simulink model "Control_APF7_nuevo_MicroLabBox"  (R2018b)
settings: Solver=FixedStepDiscrete  StartTime=0.0  StopTime=inf  FixedStep=Tm  RelTol=1e-3
PostLoadFcn:
  | , if any(exist('dsrtsu_mdlpostloadfcn', 'file') == [2, 3, 6]), try dsrtsu_mdlpostloadfcn('Execute', bdroot); catch fprintf('Error in PostLoadFcn (dsrtsu_mdlpostloadfcn) for model "%s":\n %s\n', bdroot, lasterr); end, end,
values from neighbouring files (symbols this model uses):
  e = den(1)    [parametrosAPF_nuevo.m]
  f = den(2)    [parametrosAPF_nuevo.m]
  g = den(3)    [parametrosAPF_nuevo.m]
  Ganancia_Ica = 2.6804*K    (= 26.804)    [parametrosAPF_nuevo.m]
  Ganancia_Icb = 2.7956*K    (= 27.956)    [parametrosAPF_nuevo.m]
  Ganancia_Icc = 2.7659*K    (= 27.659)    [parametrosAPF_nuevo.m]
  Ganancia_Ila = 2.7659*K    (= 27.659)    [parametrosAPF_nuevo.m]
  Ganancia_Ilb = 2.7659*K    (= 27.659)    [parametrosAPF_nuevo.m]
  Ganancia_Ilc = 2.7083*K    (= 27.083)    [parametrosAPF_nuevo.m]
  Ganancia_Vsa = 250.0    (= 250)    [parametrosAPF_nuevo.m]
  Ganancia_Vsb = 250.0    (= 250)    [parametrosAPF_nuevo.m]
  Ganancia_Vsc = 250.0    (= 250)    [parametrosAPF_nuevo.m]
  Ica_offset = 0.0    (= 0)    [parametrosAPF_nuevo.m]
  Icb_offset = 0.0    (= 0)    [parametrosAPF_nuevo.m]
  Icc_offset = 0.0    (= 0)    [parametrosAPF_nuevo.m]
  Ila_offset = 0.0    (= 0)    [parametrosAPF_nuevo.m]
  Ilb_offset = 0.0    (= 0)    [parametrosAPF_nuevo.m]
  Ilc_offset = 0.0    (= 0)    [parametrosAPF_nuevo.m]
  ki = 0.006    [parametrosAPF_nuevo.m]
  kp = 0.007    [parametrosAPF_nuevo.m]
  lamda = 0.02    [parametrosAPF_nuevo.m]
  Lc = 10e-3    (= 0.01)    [parametrosAPF_nuevo.m]
  Rc = 0.35    [parametrosAPF_nuevo.m]
  sat = 0    [parametrosAPF_nuevo.m]
  Ts = 1/10000    (= 0.0001)    [parametros.m]    (also in parametrosAPF_nuevo.m = 5.55555555556e-05)
  Vdc = 63.0    (= 63)    [parametrosAPF_nuevo.m]
  Vsa_offset = 1.507    [parametrosAPF_nuevo.m]
  Vsb_offset = 1.466    [parametrosAPF_nuevo.m]
  Vsc_offset = 1.495    [parametrosAPF_nuevo.m]
  x = num(1)    [parametrosAPF_nuevo.m]
  y = num(2)    [parametrosAPF_nuevo.m]
  z = num(3)    [parametrosAPF_nuevo.m]
libraries: rti1202lib_dio_class1 x20, rti1202lib_adc_class1 x12, RTITaskLibDemoLibInfo x2, simulink x1, rtitasklib x1
(part 1 of 4)
PreSaveFcn:
  | , if any(exist('dsmpb_private', 'file') == [2, 3, 6]), try, dsmpb_private('dsmpb_mdlclblib', 'PreSave', bdroot); catch, disp(lasterr); end, end,
CloseFcn:
  | , if any(exist('dsmpb_private', 'file') == [2, 3, 6]), try, dsmpb_private('dsmpb_mdlclblib', 'Close', bdroot); catch, disp(lasterr); end, end,
settings Model: DSRTSU_INTERNAL_RTI_VER=520  DSRTSU_INTERNAL_RTI_TYPE=rti1202  RTICANMMDATA=struct('GeneralSetupData',struct('modelroot',['C:\Users\DELL\Documents\Espinoza\APF 7Nuevo\Plantilla_Control_DMC_MicroLabBox'],'generalsettings',struct('filesettings',struct('destfolder',struct('Name','RTICANMM_FILES','Check',1),'buildfolder',struct('Name','.','Check',1),'AbsDestfolder',struct('Name',['C:\Users\DELL\Documents\Espinoza\APF 7Nuevo\Plantilla_Control_DMC_MicroLabBox\RTICANMM_FILES']),'AbsBuildfolder',struct('Name',['C:\Users\DELL\Documents\Espinoza\APF 7Nuevo\Plantilla_Control_DMC_MicroLabBox']))),'options',struct('addpaths',1,'rmpaths',1,'addtrcexclusion',logical(1),'cannavigator',struct('checkmonitoring',0),'show_usrtrc',0,'use_usrtrc',0),'advanced',struct('options',[1 1 1 1 1 1 1 1 1 1 1 1 1 1 1 1 1 1 1 1 1 1 1 1 1 1 1 1 1 1 1 1 1 1 1 1 1 1 1 1 1 1 1 1 1 1 1 1 1 1 1 1 1 1 1 1 1 1 1 1 1 1 1 1 1 1 1 1 1 1 1 1 1 1 1 1 1 1 1 1 1 1 1 1 1 1 1 1 1 1 1 1 1 1 1 1 1 1 1 1]),'MPSetup',{{}},'modelname','Control_APF7_nuevo_MicroLabBox','block','Control_APF7_nuevo_MicroLabBox'))  DSRTSU_INTERNAL_RTIFLEXRAYCONFIG=110  DSRTSU_INTERNAL_RTIFPGA=110  DSMPB_DATASERVER_ModelPortLibVersion1=8  DSMPB_DATASERVER_DataServerVersion1=6  DSMPB_DATASERVER_DataServerStreamVersion1=3  Creator=DELL  LastModifiedBy=DELL
settings OptimizationCC: BlockReduction=off  BufferReuse=off
settings HardwareCC: ProdBitPerPointer=32  ProdBitPerSizeT=32  ProdBitPerPtrDiffT=32  ProdLargestAtomicInteger=Integer  ProdEndianess=BigEndian  ProdWordSize=32  ProdHWDeviceType=Custom Processor->Custom  TargetIntDivRoundTo=Zero  TargetEndianess=BigEndian  TargetHWDeviceType=Custom Processor->Custom
settings SFSimCC: MATLABDynamicMemAlloc=off
settings RTWCC: SystemTargetFile=rti1202.tlc  MakeCommand=make_rti  TemplateMakefile=rti1202.tmf  Description=dSPACE DS1202 Hardware Platform
settings STFCustomTargetCC: ParMdlRefBuildCompliant=on  SystemTargetFile=rti1202.tlc
settings GRTTargetCC: TargetLangStandard=C89/C90 (ANSI)  CompOptLevelCompliant=off  ConcurrentExecutionCompliant=off  CombineOutputUpdateFcns=off  MatFileLogging=off  CPPClassGenCompliant=off  UseToolchainInfoCompliant=off  RTWCAPISignals=on

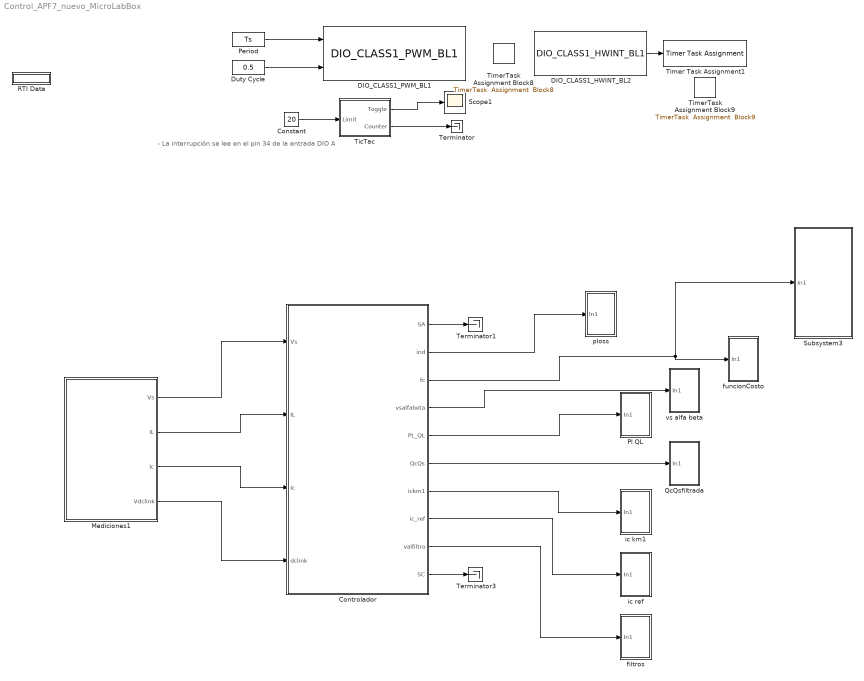
== system Control_APF7_nuevo_MicroLabBox ==
  note: - La interrupción se lee en el pin 34 de la entrada DIO A
  Constant : Constant  Value=20
  Controlador : Subsystem
  DIO_CLASS1_HWINT_BL2 : rti1202lib_dio_class1/DIO_CLASS1_HWINT_BL1  DSProperties=struct('RTI',struct('Version',uint32(2),'BlockType',struct('isSLSource',uint8(1),'isSLSink',uint8(0),'isHWSource',uint8(0),'isHWSink',uint8(0),'isSetup',uint8(0),'isInline',uint8(1),'isNonInline',uint8(0),'isInterrupt',uint8(1),'isChannelwise',uint8(0)),'IOBoardType',{{'DS120X','STD','DIOC1'}},'UnitType','DSTASKTOOL','Identifier','HWINT','DialogType','ML','BlockSet','NONE','SlaveProcessor','NONE'))  RTIBlockInterface=struct('OutputPortsActive',1,'OutputPortsWidth',int32(1),'OutputPortsName',{{'Interrupt'}},'FunctionCall',uint32(0),'DialogFcn','rti120xstddioc1hwintgui','InitLevel',3,'BlockDisplay',{{['DIO CL1 HWINT\nIdentifier: PWM\nPort: 3\nChannel: 1\nInterrupt: Falling edge'],'center'}},'IconTransparency','on','BlockName',struct('Token',{{'DIO_CLASS1_HWINT_BL1'}}))  RTIBlockParameters=struct('SourceBlockListIdx',{{2,'OFF',[1 2]}},'SourceBlockIdentifier',{{'PWM','OFF',[]}},'InterruptTypeListIdx',{{2,'OFF',[1 2]}},'InterruptType',{{['Falling edge'],'OFF',[]}},'PortNo',{{3,'OFF',[]}},'ChannelNo',{{1,'OFF',[]}})  RTISFcnParameters=struct('PortNo','int16','ChannelNo','int16')  RTIBlockParaDefault=struct('SourceBlockListIdx',1,'SourceBlockIdentifier',['NOT SELECTED'],'InterruptTypeListIdx',1,'InterruptType',['NOT SELECTED'],'PortNo',-1,'ChannelNo',-1)
  DIO_CLASS1_PWM_BL1 : rti1202lib_dio_class1/DIO_CLASS1_PWM_BL1  DSProperties=struct('RTI',struct('Version',uint32(1),'BlockType',struct('isSLSource',uint8(0),'isSLSink',uint8(1),'isHWSource',uint8(0),'isHWSink',uint8(1),'isSetup',uint8(0),'isInline',uint8(1),'isNonInline',uint8(0),'isInterrupt',uint8(0),'isChannelwise',uint8(1)),'IOBoardType',{{'DS120X','STD','DIOC1'}},'UnitType','PWM','Identifier','PWM','DialogType','ML','BlockSet','NONE','SlaveProcessor','NONE'))  RTIBlockInterface=struct('InputPortsWidth',int32([1 1]),'InputPortsActive',[1 1],'InputPortsName',{{'Period',['Duty Cycle']}},'BlockDisplay',{{['DIO CL1 PWM\nPort: 3\nChannel: 1'],'center'}},'IconTransparency','on','InitLevel',3,'DialogFcn','rti120xstddioc1pwmgui','BlockName',struct('Token',{{'DIO_CLASS1_PWM_BL1'}}))  RTIBlockParameters=struct('PortNo',{{3,'OFF',[]}},'ChannelNo',{{1,'OFF',[]}},'HighLevel',{{3,'OFF',[1 3]}},'UpdateMode',{{2,'OFF',[1 2]}},'InvertingMode',{{1,'OFF',[1 2]}},'DutyCycleInit',{{'0.5','OFF',[0 1]}},'DutyCycleTerm',{{'0.5','OFF',[0 1]}},'PeriodInit',{{'5e-05','OFF',[1e-7 1.34]}},'PeriodTerm',{{'5e-05','OFF',[1e-7 1.34]}},'TerminationMode',{{0,'OFF',[0 1]}},'OutputTermValidate',{{0,'OFF',[0 1]}},'OutputTermBuildCheck',{{logical(0),'OFF',[]}},'EnableEvent',{{1,'OFF',[0 1]}},'EventMode',{{1,'OFF',[1 3]}},'EventOnFalling',{{1,'OFF',[0 1]}},'EventOnRising',{{0,'OFF',[0 1]}},'EventDelay',{{'0','OFF',[0 1.34]}},'EventRate',{{'1','OFF',[1 256]}},'EventBuildCheck',{{logical(1),'OFF',[]}},'TriggerLine',{{1,'OFF',[1 16]}},'TLCFileName',{{'rti120xdio_c1_pwm','OFF',[]}})  RTISFcnParameters=struct('PortNo','int16','ChannelNo','int16','HighLevel','int16','UpdateMode','int16','InvertingMode','int16','DutyCycleInit','double','DutyCycleTerm','double','PeriodInit','double','PeriodTerm','double','TerminationMode','int16','OutputTermValidate','int16','EnableEvent','int16','EventMode','int16','EventOnFalling','int16','EventOnRising','int16','EventDelay','double','EventRate','int16','TriggerLine','int16','TLCFileName','char')  RTIBlockParaDefault=struct('PortNo',1,'ChannelNo',1,'HighLevel',1,'UpdateMode',1,'InvertingMode',1,'DutyCycleInit',2^-1,'DutyCycleTerm',2^-1,'PeriodInit',5e-5,'PeriodTerm',5e-5,'TerminationMode',0,'OutputTermValidate',0,'OutputTermBuildCheck',0,'EnableEvent',0,'EventMode',1,'EventOnFalling',1,'EventOnRising',0,'EventDelay',0,'EventRate',1,'EventBuildCheck',0,'TriggerLine',1,'TLCFileName','rti120xdio_c1_pwm')
  Duty Cycle : Constant  Value=0.5
  Mediciones1 : Subsystem
  Period : Constant  Value=Ts
  "Pl QL " : Subsystem
  QcQsfiltrada : Subsystem
  RTI Data : Subsystem  Tag=struct('RTIDataServer',struct('RTIDataServerVs','2','RTIModelDescription','struct(''main'',''Control_APF7_nuevo_MicroLabBox'',''sub'','''',''isMp'',0)'))  LoadFcn="if exist('rtidc'), try,  rtidc('DataHostBlockClbLoad', gcbh); catch, disp(['Warning: ''LoadFcn'' for RTI Data block failed: ' lasterr]); end, end,"  mask(RTI_DATA_HOST){}
      mask help:
      | RTI Data Block.
      | This block is used by RTI to store internal model-dependent data.
      | Please keep this block on the root level of the model. Deleting this block will result in data loss.
      |
      | NEVER DELETE OR COPY THIS BLOCK!
      settings: CopyFcn="if exist('rtidc'), try,  rtidc('DataHostBlockClbCopy', gcbh); catch, disp(['Warning: ''CopyFcn'' for RTI Data block failed: ' lasterr]); end, end,"  DeleteFcn="if exist('rtidc'), try,  rtidc('DataHostBlockClbDelete', gcbh); catch, disp(['Warning: ''DeleteFcn'' for RTI Data block failed: ' lasterr]); end, end,"  ModelCloseFcn="if exist('rtidc'), try,  rtidc('DataHostBlockClbModelClose', gcbh); catch, disp(['Warning: ''ModelCloseFcn'' for RTI Data block failed: ' lasterr]); end, end,"  PreSaveFcn="if exist('rtidc'), try,  rtidc('DataHostBlockClbPreSave', gcbh); catch, disp(['Warning: ''PreSaveFcn'' for RTI Data block failed: ' lasterr]); end, end,"  PostSaveFcn="if exist('rtidc'), try,  rtidc('DataHostBlockClbPostSave', gcbh); catch, disp(['Warning: ''PostSaveFcn'' for RTI Data block failed: ' lasterr]); end, end,"  NameChangeFcn="if exist('rtidc'), try,  rtidc('DataHostBlockClbNameChange', gcbh); catch, disp(['Warning: ''NameChangeFcn'' for RTI Data block failed: ' lasterr]); end, end,"
      mask Help:
      | RTI Data Block.
      | This block is used by RTI to store internal model-dependent data.
      | Please keep this block on the root level of the model. Deleting this block will result in data loss.
      | 
      | NEVER DELETE OR COPY THIS BLOCK!
      mask Display:
      | text(0.5, 0.5, 'RTI Data', 'HorizontalAlignment', 'center');
      | plot([1 0]);
  Scope1 : Scope
  Subsystem3 : Subsystem
  Terminator : Terminator
  Terminator1 : Terminator
  Terminator3 : Terminator
  TicTac : Subsystem
      mask help:
      | The output "Toggle" changes its output between -1 and 1 each time the block is executed.
      |
      | The output "Counter" counts up to the given "Limit" and then resets to one.
  Timer Task Assignment1 : rtitasklib/Timer Task Assignment  Reserved2=[]  Reserved3=[]  Reserved4=[]  DSProperties=struct('RTI',struct('Version',uint32(2),'BlockType',struct('isSLSource',uint8(0),'isSLSink',uint8(1),'isHWSource',uint8(0),'isHWSink',uint8(0),'isSetup',uint8(0),'isInline',uint8(1),'isNonInline',uint8(0),'isInterrupt',uint8(0),'isChannelwise',uint8(0)),'IOBoardType','INTLIB','UnitType','TTASSIGN','Identifier','TTASSIGN','DialogType','SL','BlockSet','NONE','SlaveProcessor','NONE','RelationId',struct('TH',struct('BlockId','TTASSIGN'))))
  TimerTask Assignment Block8 : RTITaskLibDemoLibInfo/TimerTask  Assignment  Block8  SystemSampleTime=-1
  TimerTask Assignment Block9 : RTITaskLibDemoLibInfo/TimerTask  Assignment  Block9  SystemSampleTime=-1
  filtros : Subsystem
  "funcionCosto " : Subsystem
  "ic km1 " : Subsystem
  "ic ref " : Subsystem
  ploss : Subsystem
  "vs alfa beta " : Subsystem
  wires:
  Mediciones1/2(IL) -> Controlador/2(IL)
  Mediciones1/3(Ic) -> Controlador/3(Ic)
  TicTac/1(Toggle) -> Scope1/1
  Constant/1 -> TicTac/1(Limit)
  DIO_CLASS1_HWINT_BL2/1 -> Timer Task Assignment1/1
  Period/1 -> DIO_CLASS1_PWM_BL1/1
  Duty Cycle/1 -> DIO_CLASS1_PWM_BL1/2
  TicTac/2(Counter) -> Terminator/1
  Controlador/4(vsalfabeta) -> "vs alfa beta "/1(In1)
  Controlador/6(QcQs) -> QcQsfiltrada/1(In1)
  Controlador/5(PL_QL) -> "Pl QL "/1(In1)
  Controlador/8(ic_ref) -> "ic ref "/1(In1)
  Controlador/7(ickm1) -> "ic km1 "/1(In1)
  Controlador/1(SA) -> Terminator1/1
  Controlador/9(valfiltro) -> filtros/1(In1)
  Controlador/10(SC) -> Terminator3/1
  Controlador/3(fc) -> Subsystem3/1(In1), "funcionCosto "/1(In1)
  Controlador/2(ind) -> ploss/1(In1)
  Mediciones1/4(Vdclink) -> Controlador/4(dclink)
  Mediciones1/1(Vs) -> Controlador/1(Vs)

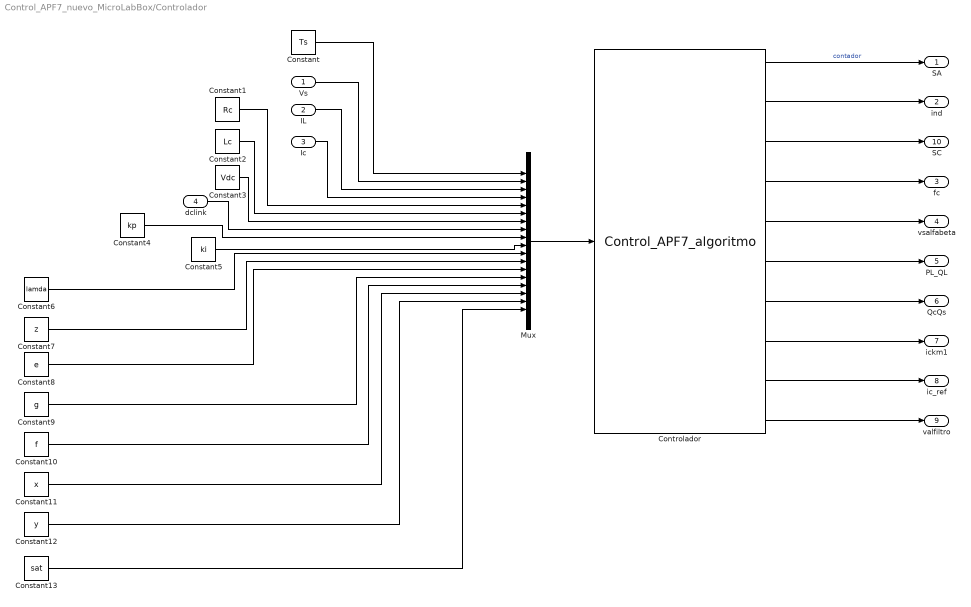
== system Control_APF7_nuevo_MicroLabBox/Controlador ==
  Vs : Inport
  IL : Inport  Port=2
  Ic : Inport  Port=3
  dclink : Inport  Port=4
  Constant : Constant  Value=Ts
  Constant1 : Constant  Value=Rc
  Constant10 : Constant  Value=f
  Constant11 : Constant  Value=x
  Constant12 : Constant  Value=y
  Constant13 : Constant  Value=sat
  Constant2 : Constant  Value=Lc
  Constant3 : Constant  Value=Vdc
  Constant4 : Constant  Value=kp
  Constant5 : Constant  Value=ki
  Constant6 : Constant  Value=lamda
  Constant7 : Constant  Value=z
  Constant8 : Constant  Value=e
  Constant9 : Constant  Value=g
  Controlador : S-Function  InitFcn=try, set_param(gcb,'FunctionName','Control_APF7_algoritmo'), end  FunctionName=Control_APF7_algoritmo  SFunctionModules=Control_APF7_algoritmo_wrapper  SFunctionDeploymentMode=off  EnableBusSupport=off  mask(S-Function Builder){}
      mask help: Simulink:masks:SFunctionBuilder_MD
      mask init:
      | val = [[.9  0.75 0.75 1 1 .9 .9 1]',[1 1 0.75 0.75 .9 .9 1 .9]'];try , sys = get_param(gcb,'SfunBuilderFcnName');if isempty(sys), sys = get_param(gcb,'FunctionName'); end,catch, sys = get_param(gcb,'FunctionName'); end
      settings: CopyFcn=set_param(gcbh,'LinkStatus','none')  PreSaveFcn=try, set_param(gcb,'FunctionName','Control_APF7_algoritmo'), end  OpenFcn=sfunctionwizard(gcbh)
      mask Display: plot(val(:,1),val(:,2)),disp(sys), port_label('input',1,'in'), port_label('output',1,'SwA'), port_label('output',2,'io'), port_label('output',3,'SwC'), port_label('output',4,'fc'), port_label('output',5,'Vs_alfabeta'), port_label('output',6,'PLQL'), port_label('output',7,'QCQS'), port_label('output',8,'ic_km1'), port_label('output',9,'Icref'), port_label('output',10,'Varfiltro')
  Mux : Mux  Inputs=18
  SA : Outport
  ind : Outport  Port=2
  fc : Outport  Port=3
  vsalfabeta : Outport  Port=4
  PL_QL : Outport  Port=5
  QcQs : Outport  Port=6
  ickm1 : Outport  Port=7
  ic_ref : Outport  Port=8
  valfiltro : Outport  Port=9
  SC : Outport  Port=10
  wires:
  Constant3/1 -> Mux/7
  Constant1/1 -> Mux/5
  IL/1 -> Mux/3
  Ic/1 -> Mux/4
  Constant/1 -> Mux/1
  Constant2/1 -> Mux/6
  Mux/1 -> Controlador/1
  dclink/1 -> Mux/8
  Controlador/8 -> ickm1/1
  Vs/1 -> Mux/2
  Controlador/3 -> SC/1
  Controlador/2 -> ind/1
  Controlador/1 -> SA/1  "contador"
  Controlador/4 -> fc/1
  Controlador/6 -> PL_QL/1
  Controlador/5 -> vsalfabeta/1
  Controlador/7 -> QcQs/1
  Controlador/10 -> valfiltro/1
  Controlador/9 -> ic_ref/1
  Constant4/1 -> Mux/9
  Constant5/1 -> Mux/10
  Constant6/1 -> Mux/11
  Constant7/1 -> Mux/12
  Constant8/1 -> Mux/13
  Constant9/1 -> Mux/14
  Constant10/1 -> Mux/15
  Constant11/1 -> Mux/16
  Constant12/1 -> Mux/17
  Constant13/1 -> Mux/18
